simulink model "p4"  (R2021b)
settings: Solver=VariableStepAuto  StartTime=0.0  StopTime=100  RelTol=1e-3
settings Model: Creator=hp  LastModifiedBy=hp

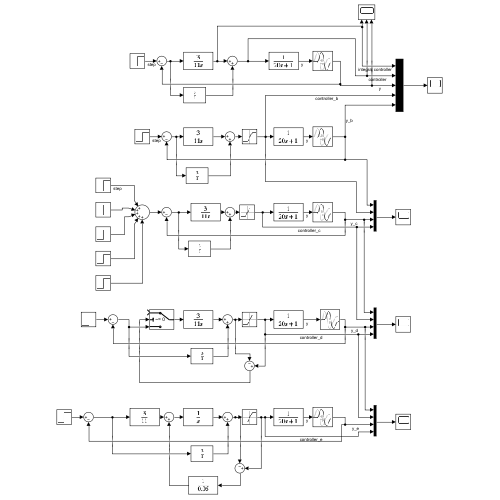
[thumbnail: Simulink's stored preview of the top-level diagram]
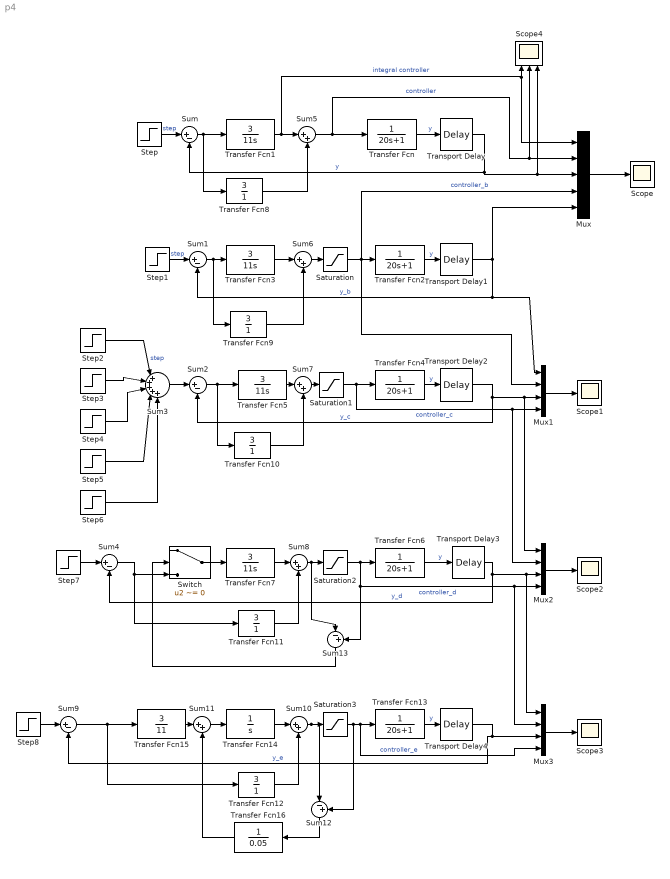
== system p4 ==
  Mux : Mux  Inputs=5
  Mux1 : Mux
  Mux2 : Mux
  Mux3 : Mux
  Saturation{,1..3} (4 alike) : Saturate  UpperLimit=2  LowerLimit=-2
  Scope{,1..3} (4 alike) : Scope
  Scope4 : Scope  NumInputPorts=3
  Step{,1,7..8} (4 alike) : Step  Time=0  SampleTime=0
  Step2 : Step  Time=0  After=0.2  SampleTime=0
  Step3 : Step  Time=5  After=0.2  SampleTime=0
  Step4 : Step  Time=10  After=0.2  SampleTime=0
  Step5 : Step  Time=15  After=0.2  SampleTime=0
  Step6 : Step  Time=20  After=0.2  SampleTime=0
  Sum{,1..2,4,9} (5 alike) : Sum  Inputs=|+-
  Sum{5..8,10..11} (6 alike) : Sum  Inputs=|++
  Sum12 : Sum  Inputs=|-+
  Sum13 : Sum  Inputs=|-+
  Sum3 : Sum  Inputs=|+++++
  Switch : Switch  Criteria=u2 ~= 0
  Transfer Fcn{,2,4,6,13} (5 alike) : TransferFcn  Denominator=[20 1]
  Transfer Fcn{1,3,5,7} (4 alike) : TransferFcn  Numerator=[3]  Denominator=[11 0]
  Transfer Fcn{8..12} (5 alike) : TransferFcn  Numerator=[3]  Denominator=[1]
  Transfer Fcn14 : TransferFcn  Denominator=[1 0]
  Transfer Fcn15 : TransferFcn  Numerator=[3]  Denominator=[11]
  Transfer Fcn16 : TransferFcn  Denominator=[0.05]
  Transport Delay{,1..4} (5 alike) : TransportDelay  DelayTime=4
  wires:
  Transfer Fcn/1 -> Transport Delay/1  "y"
  Step/1 -> Sum/1  "step"
  Saturation/1 -> Mux1/2, Mux/4, Transfer Fcn2/1  "controller_b"
  Sum/1 -> Transfer Fcn8/1, Transfer Fcn1/1
  Transport Delay/1 -> Mux/3, Scope4/3, Sum/2  "y"
  Transfer Fcn2/1 -> Transport Delay1/1  "y"
  Step1/1 -> Sum1/1  "step"
  Transport Delay1/1 -> Mux1/1, Sum1/2, Mux/5  "y_b"
  Transfer Fcn4/1 -> Transport Delay2/1  "y"
  Sum3/1 -> Sum2/1
  Step2/1 -> Sum3/1  "step"
  Step3/1 -> Sum3/2
  Step4/1 -> Sum3/3
  Step5/1 -> Sum3/4
  Step6/1 -> Sum3/5
  Mux1/1 -> Scope1/1
  Mux/1 -> Scope/1
  Transport Delay3/1 -> Mux3/1, Mux2/3, Sum4/2  "y_d"
  Saturation2/1 -> Sum13/2, Mux3/2, Mux2/4, Transfer Fcn6/1  "controller_d"
  Transfer Fcn6/1 -> Transport Delay3/1  "y"
  Saturation1/1 -> Transfer Fcn4/1, Mux2/2, Mux1/4  "controller_c"
  Mux2/1 -> Scope2/1
  Transport Delay2/1 -> Mux2/1, Mux1/3, Sum2/2  "y_c"
  Step7/1 -> Sum4/1
  Transfer Fcn1/1 -> Mux/1, Scope4/1, Sum5/1  "integral controller"
  Sum5/1 -> Mux/2, Scope4/2, Transfer Fcn/1  "controller"
  Transfer Fcn8/1 -> Sum5/2
  Transfer Fcn3/1 -> Sum6/1
  Sum6/1 -> Saturation/1
  Transfer Fcn9/1 -> Sum6/2
  Sum1/1 -> Transfer Fcn9/1, Transfer Fcn3/1
  Sum7/1 -> Saturation1/1
  Transfer Fcn5/1 -> Sum7/1
  Sum2/1 -> Transfer Fcn10/1, Transfer Fcn5/1
  Transfer Fcn10/1 -> Sum7/2
  Transfer Fcn7/1 -> Sum8/1
  Sum8/1 -> Sum13/1, Saturation2/1
  Sum4/1 -> Switch/3, Transfer Fcn11/1
  Transfer Fcn11/1 -> Sum8/2
  Switch/1 -> Transfer Fcn7/1
  Transfer Fcn14/1 -> Sum10/1
  Sum10/1 -> Sum12/1, Saturation3/1
  Sum9/1 -> Transfer Fcn15/1, Transfer Fcn12/1
  Saturation3/1 -> Sum12/2, Mux3/4, Transfer Fcn13/1  "controller_e"
  Mux3/1 -> Scope3/1
  Transfer Fcn13/1 -> Transport Delay4/1  "y"
  Transfer Fcn12/1 -> Sum10/2
  Transport Delay4/1 -> Mux3/3, Sum9/2  "y_e"
  Step8/1 -> Sum9/1
  Sum11/1 -> Transfer Fcn14/1
  Transfer Fcn15/1 -> Sum11/1
  Transfer Fcn16/1 -> Sum11/2
  Sum12/1 -> Transfer Fcn16/1
  Sum13/1 -> Switch/2
